simulink model "normModel"  (Simulink 7.7)
settings: Solver=ode45  StartTime=0.0  StopTime=10.0  RelTol=1e-3
values from neighbouring files (symbols this model uses):
  Am = 0    [Vndr8wGKHogMolcBQBjUJcBv5rTWana5.m]
  NP = 0.5    [Vndr8wGKHogMolcBQBjUJcBv5rTWana5.m]
  R = b    [Vndr8wGKHogMolcBQBjUJcBv5rTWana5.m]
  to = randseed    [Vndr8wGKHogMolcBQBjUJcBv5rTWana5.m]
  Ts = 0.001    [Vndr8wGKHogMolcBQBjUJcBv5rTWana5.m]
libraries: commanapbnd3 x2
settings Model: Creator=Enko  LastModifiedBy=Enko
settings DebuggingCC: SolverPrmCheckMsg=none

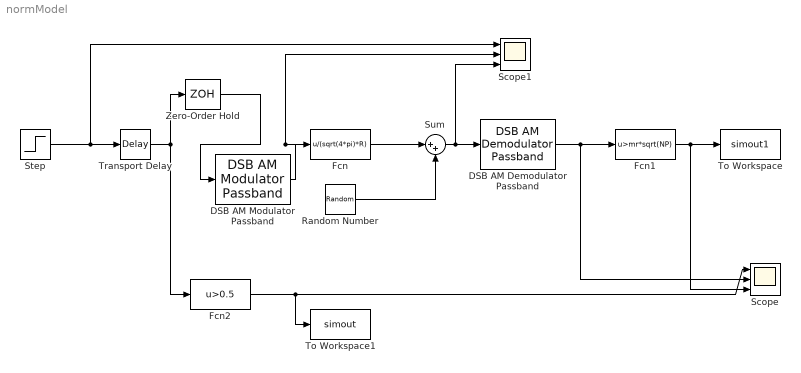
== system normModel ==
  DSB AM Demodulator Passband : commanapbnd3/DSB AM Demodulator Passband  SystemSampleTime=-1  Fc=1000  Ph=0  method=Butterworth  n=4  cf=1  Rp=0.1  Rs=50  Offset=0
  DSB AM Modulator Passband : commanapbnd3/DSB AM Modulator Passband  SystemSampleTime=-1  Fc=1000  Ph=0  Offset=0
  Fcn : Fcn  Expr=u/(sqrt(4*pi)*R)  SampleTime=Ts
  Fcn1 : Fcn  Expr=u>mr*sqrt(NP)  SampleTime=Ts
  Fcn2 : Fcn  Expr=u>0.5  SampleTime=Ts
  Random Number : RandomNumber  Variance=NP  Seed=to  SampleTime=Ts
  Scope : Scope  NumInputPorts=3
      settings: YMin=-5~-5~-5  YMax=5~5~5
  Scope1 : Scope  NumInputPorts=3
      settings: YMin=-5~-5~-5  YMax=5~5~5
  Step : Step  Before=Am  After=0  SampleTime=Ts
  Sum : Sum  Inputs=|++
  To Workspace : ToWorkspace  VariableName=simout1  SampleTime=1  SaveFormat=Array
  To Workspace1 : ToWorkspace  VariableName=simout  SampleTime=1  SaveFormat=Array
  Transport Delay : TransportDelay  DelayTime=4.5  BufferSize=10240
  Zero-Order Hold : ZeroOrderHold  SampleTime=Ts
  wires:
  Step/1 -> Transport Delay/1, Scope1/1
  Transport Delay/1 -> Fcn2/1, Zero-Order Hold/1
  Random Number/1 -> Sum/2
  DSB AM Modulator Passband/1 -> Fcn/1, Scope1/2
  Fcn/1 -> Sum/1
  Sum/1 -> DSB AM Demodulator Passband/1, Scope1/3
  DSB AM Demodulator Passband/1 -> Fcn1/1, Scope/2
  Fcn1/1 -> To Workspace/1, Scope/3
  Fcn2/1 -> To Workspace1/1, Scope/1
  Zero-Order Hold/1 -> DSB AM Modulator Passband/1
